simulink model "fir_multi_test"  (Simulink 7.8)
settings: Solver=ode45  StartTime=0.0  StopTime=15e-4  RelTol=1e-3
undefined symbols (not defined in the file): calc_dds_freq, Fs_adc, Fs_adc_image, xlipgetpartsetting
libraries: xbsIndex_r4 x24
settings Model: Creator=lucas.russo  LastModifiedBy=lucas.russo

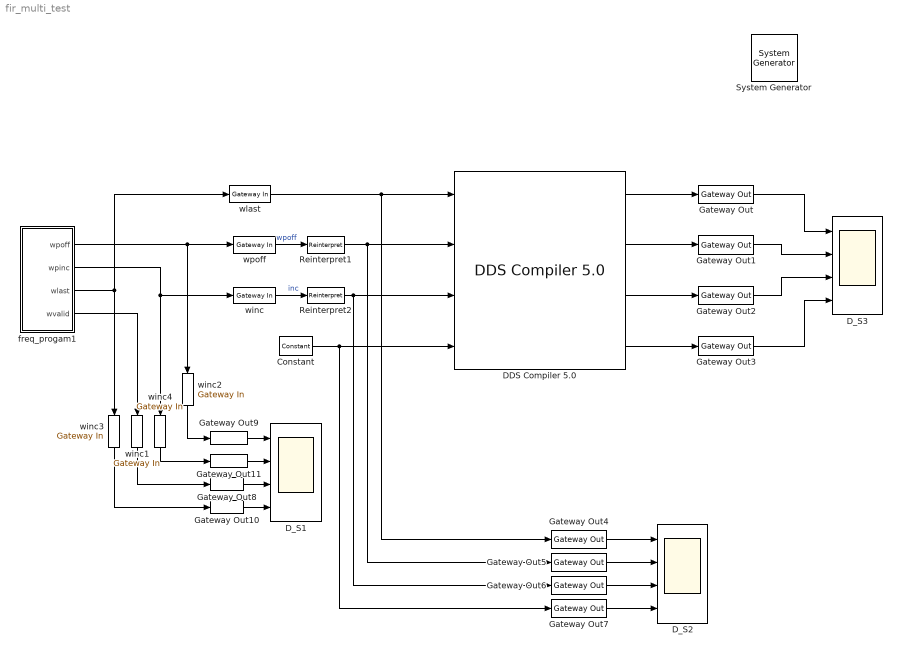
== system fir_multi_test ==
  " System Generator" : xbsIndex_r4/ System Generator  Tag=genX  xilinxfamily=virtex6  part=xc6vlx240t  speed=-1  package=ff1156  synthesis_tool=XST  clock_wrapper=Clock Enables  directory=./netlist  proj_type=Project Navigator  Synth_file=XST Defaults  Impl_file=ISE Defaults  testbench=off  simulink_period=dt_sim  sysclk_period=20  dcm_input_clock_period=10  incr_netlist=off  trim_vbits=Everywhere in SubSystem  dbl_ovrd=According to Block Masks  core_generation=According to Block Masks  run_coregen=off  deprecated_control=off  eval_field=0  block_type=sysgen
  Constant : xbsIndex_r4/Constant  const=1  gui_display_data_type=Boolean  arith_type=Boolean  n_bits=1  bin_pt=0  preci_type=Single  exp_width=8  frac_width=24  explicit_period=on  period=dt_sim  equ=P=C  opselect=C  inp2=PCIN>>17  opr=+  inp1=P  carry=CIN  dbl_ovrd=off  block_type=constant
  DDS Compiler 5.0 : xbsIndex_r4/DDS Compiler 5.0   partspresent=Phase_Generator_and_SIN_COS_LUT  dds_clock_rate=Fs_adc/1e6  channels=1  parameter_entry=Hardware_Parameters  spurious_free_dynamic_range=36  frequency_resolution=0.4  noise_shaping=Taylor_Series_Corrected  phase_width=30  output_width=24  output_selection=Sine_and_Cosine  negative_sine=on  negative_cosine=off  amplitude_mode=Unit_Circle  memory_type=Auto  optimization_goal=Auto  dsp48_use=Minimal  latency_configuration=Auto  latency=14  has_phase_out=off  has_aclken=off  has_aresetn=off  explicit_period=on  period=dt_sim  data_has_tlast=Not_Required  has_tready=on  s_phase_has_tuser=Not_Required  m_data_has_tuser=Not_Required  m_phase_has_tuser=Not_Required  s_phase_tuser_width=1  s_config_sync_mode=On_Vector  phase_increment=Programmable  output_frequency1=0  output_frequency2=0  output_frequency3=0  output_frequency4=0  output_frequency5=0  output_frequency6=0  output_frequency7=0  output_frequency8=0  output_frequency9=0  output_frequency10=0  output_frequency11=0  output_frequency12=0  output_frequency13=0  output_frequency14=0  output_frequency15=0  output_frequency16=0  pinc1='0'  pinc2='0'  pinc3='0'  pinc4='0'  pinc5='0'  pinc6='0'  pinc7='0'  pinc8='0'  pinc9='0'  pinc10='0'  pinc11='0'  pinc12='0'  pinc13='0'  pinc14='0'  pinc15='0'  pinc16='0'  phase_offset=Programmable  phase_offset_angles1=0  phase_offset_angles2=0  phase_offset_angles3=0  phase_offset_angles4=0  phase_offset_angles5=0  phase_offset_angles6=0  phase_offset_angles7=0  phase_offset_angles8=0  phase_offset_angles9=0  phase_offset_angles10=0  phase_offset_angles11=0  phase_offset_angles12=0  phase_offset_angles13=0  phase_offset_angles14=0  phase_offset_angles15=0  phase_offset_angles16=0  poff1='0'  poff2='0'  poff3='0'  poff4='0'  poff5='0'  poff6='0'  poff7='0'  poff8='0'  poff9='0'  poff10='0'  poff11='0'  poff12='0'  poff13='0'  poff14='0'  poff15='0'  poff16='0'  trim_axipin_name=on  por_mode=false  gui_behaviour=Sysgen  ip_name=DDS Compiler  ip_version=5.0  dsptool_ready=true  wrapper_available=true  port_translation_map={ 'aclken' => 'en', 'aresetn' => 'rst' }  ipcore_xco_need_fpga_part=true  ipcore_fpga_part=xlipgetpartsetting(gcb, {'virtex6', 'xc6vlx75t', '-3', 'ff784'})  ipcore_usecache=true  ipcore_useipmodelcache=true  ipcore_verbose=false  block_type=dds_compiler_v5_0
  D_S1 : Scope  NumInputPorts=4
      settings: TimeRange=0.0004  YMin=0.95~0.95~-1~0.95  YMax=1.05~1.05~1~1.05  MaxDataPoints=1000000  SampleInput=on
  D_S2 : Scope  NumInputPorts=4
      settings: TimeRange=0.0004  YMin=0.95~0.95~-1~0.95  YMax=1.05~1.05~1~1.05  SaveName=ScopeData2  MaxDataPoints=1000000  SampleInput=on
  D_S3 : Scope  NumInputPorts=4
      settings: TimeRange=0.0004  YMin=1~1~-1~1  YMax=1~1~1~1  MaxDataPoints=1000000  SampleInput=on
  Gateway Out{,1..11} (12 alike) : xbsIndex_r4/Gateway Out  inherit_from_input=on  hdl_port=on  timing_constraint=None  locs_specified=off  LOCs={}  UseAsDAC=off  DACChannel='1'  block_type=gatewayout
      settings: infoedit="Gateway out block.  Converts Xilinx fixed-point or floating-point type inputs into ouputs of type Simulink integer, single, double, or fixed point.<br><br>Hardware notes:  In hardware these blocks become top level output ports or are discarded, depending on how they are configured."
  Reinterpret1 : xbsIndex_r4/Reinterpret  force_arith_type=off  arith_type=Unsigned  force_bin_pt=on  bin_pt=30  block_type=reinterpret
  Reinterpret2 : xbsIndex_r4/Reinterpret  force_arith_type=off  arith_type=Unsigned  force_bin_pt=on  bin_pt=30  block_type=reinterpret
  freq_progam1 : Subsystem  mask(DDS Freq. Programming Stimulus){FREQ_VEC=[ Fs_adc_image ] / 1e6, Fc=Fs_adc/1e6, Pwidth=30}
      mask prompts: FREQ_VEC "Frequency Vector (MHz)"; Fc "Sample Freq (MHz)"; Pwidth "DDS Phase Width (bits)"
      mask help: This block writes the desired mixing freqencies into the programmable frequency port of the DDS.
  winc : xbsIndex_r4/Gateway In  gui_display_data_type=Fixed-point  arith_type="Signed  (2's comp)"  n_bits=30  bin_pt=0  preci_type=Single  exp_width=8  frac_width=24  quantization=Truncate  overflow=Wrap  period=dt_sim  dbl_ovrd=off  timing_constraint=None  locs_specified=off  LOCs={}  inherit_from_input=off  UseAsADC=off  ADCChannel='1'  hdl_port=on  block_type=gatewayin
      settings: infoedit="Gateway in block.  Converts inputs of type Simulink integer, single, double and fixed point to  Xilinx fixed-point or floating-point data type.<br><br>Hardware notes:  In hardware these blocks become top level input ports."
  winc1 : xbsIndex_r4/Gateway In  gui_display_data_type=Boolean  arith_type=Boolean  n_bits=30  bin_pt=0  preci_type=Single  exp_width=8  frac_width=24  quantization=Truncate  overflow=Wrap  period=dt_sim  dbl_ovrd=off  timing_constraint=None  locs_specified=off  LOCs={}  inherit_from_input=off  UseAsADC=off  ADCChannel='1'  hdl_port=on  block_type=gatewayin
      settings: infoedit="Gateway in block.  Converts inputs of type Simulink integer, single, double and fixed point to  Xilinx fixed-point or floating-point data type.<br><br>Hardware notes:  In hardware these blocks become top level input ports."
  winc2 : xbsIndex_r4/Gateway In  gui_display_data_type=Fixed-point  arith_type="Signed  (2's comp)"  n_bits=30  bin_pt=0  preci_type=Single  exp_width=8  frac_width=24  quantization=Truncate  overflow=Wrap  period=dt_sim  dbl_ovrd=off  timing_constraint=None  locs_specified=off  LOCs={}  inherit_from_input=off  UseAsADC=off  ADCChannel='1'  hdl_port=on  block_type=gatewayin
      settings: infoedit="Gateway in block.  Converts inputs of type Simulink integer, single, double and fixed point to  Xilinx fixed-point or floating-point data type.<br><br>Hardware notes:  In hardware these blocks become top level input ports."
  winc3 : xbsIndex_r4/Gateway In  gui_display_data_type=Boolean  arith_type=Boolean  n_bits=30  bin_pt=0  preci_type=Single  exp_width=8  frac_width=24  quantization=Truncate  overflow=Wrap  period=dt_sim  dbl_ovrd=off  timing_constraint=None  locs_specified=off  LOCs={}  inherit_from_input=off  UseAsADC=off  ADCChannel='1'  hdl_port=on  block_type=gatewayin
      settings: infoedit="Gateway in block.  Converts inputs of type Simulink integer, single, double and fixed point to  Xilinx fixed-point or floating-point data type.<br><br>Hardware notes:  In hardware these blocks become top level input ports."
  winc4 : xbsIndex_r4/Gateway In  gui_display_data_type=Fixed-point  arith_type="Signed  (2's comp)"  n_bits=30  bin_pt=0  preci_type=Single  exp_width=8  frac_width=24  quantization=Truncate  overflow=Wrap  period=dt_sim  dbl_ovrd=off  timing_constraint=None  locs_specified=off  LOCs={}  inherit_from_input=off  UseAsADC=off  ADCChannel='1'  hdl_port=on  block_type=gatewayin
      settings: infoedit="Gateway in block.  Converts inputs of type Simulink integer, single, double and fixed point to  Xilinx fixed-point or floating-point data type.<br><br>Hardware notes:  In hardware these blocks become top level input ports."
  wlast : xbsIndex_r4/Gateway In  gui_display_data_type=Boolean  arith_type=Boolean  n_bits=1  bin_pt=0  preci_type=Single  exp_width=8  frac_width=24  quantization=Truncate  overflow=Wrap  period=dt_sim  dbl_ovrd=off  timing_constraint=None  locs_specified=off  LOCs={}  inherit_from_input=off  UseAsADC=off  ADCChannel='1'  hdl_port=on  block_type=gatewayin
      settings: infoedit="Gateway in block.  Converts inputs of type Simulink integer, single, double and fixed point to  Xilinx fixed-point or floating-point data type.<br><br>Hardware notes:  In hardware these blocks become top level input ports."
  wpoff : xbsIndex_r4/Gateway In  gui_display_data_type=Fixed-point  arith_type="Signed  (2's comp)"  n_bits=30  bin_pt=0  preci_type=Single  exp_width=8  frac_width=24  quantization=Truncate  overflow=Wrap  period=dt_sim  dbl_ovrd=off  timing_constraint=None  locs_specified=off  LOCs={}  inherit_from_input=off  UseAsADC=off  ADCChannel='1'  hdl_port=on  block_type=gatewayin
      settings: infoedit="Gateway in block.  Converts inputs of type Simulink integer, single, double and fixed point to  Xilinx fixed-point or floating-point data type.<br><br>Hardware notes:  In hardware these blocks become top level input ports."
  wires:
  winc/1 -> Reinterpret2/1  "inc"
  Constant/1 -> Gateway Out7/1, DDS Compiler 5.0/4
  wpoff/1 -> Reinterpret1/1  "wpoff"
  DDS Compiler 5.0/4 -> Gateway Out3/1
  DDS Compiler 5.0/3 -> Gateway Out2/1
  DDS Compiler 5.0/2 -> Gateway Out1/1
  DDS Compiler 5.0/1 -> Gateway Out/1
  Gateway Out/1 -> D_S3/1
  Gateway Out1/1 -> D_S3/2
  Gateway Out2/1 -> D_S3/3
  Gateway Out3/1 -> D_S3/4
  freq_progam1/2(wpinc) -> winc/1, winc4/1
  freq_progam1/1(wpoff) -> wpoff/1, winc2/1
  freq_progam1/3(wlast) -> wlast/1, winc3/1
  wlast/1 -> DDS Compiler 5.0/1, Gateway Out4/1
  freq_progam1/4(wvalid) -> winc1/1
  Gateway Out4/1 -> D_S2/1
  Gateway Out5/1 -> D_S2/2
  Gateway Out6/1 -> D_S2/3
  Gateway Out7/1 -> D_S2/4
  Reinterpret1/1 -> DDS Compiler 5.0/2, Gateway Out5/1
  Reinterpret2/1 -> DDS Compiler 5.0/3, Gateway Out6/1
  winc1/1 -> Gateway Out8/1
  Gateway Out8/1 -> D_S1/3
  winc2/1 -> Gateway Out9/1
  Gateway Out9/1 -> D_S1/1
  winc3/1 -> Gateway Out10/1
  Gateway Out10/1 -> D_S1/4
  Gateway Out11/1 -> D_S1/2
  winc4/1 -> Gateway Out11/1

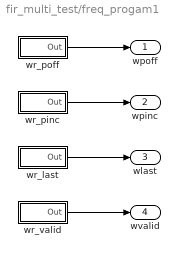
== system fir_multi_test/freq_progam1 ==
  wr_last : Subsystem
  wr_pinc : Subsystem
  wr_poff : Subsystem
  wr_valid : Subsystem
  wpoff : Outport
  wpinc : Outport  Port=2
  wlast : Outport  Port=3
  wvalid : Outport  Port=4
  wires:
  wr_last/1(Out) -> wlast/1
  wr_poff/1(Out) -> wpoff/1
  wr_pinc/1(Out) -> wpinc/1
  wr_valid/1(Out) -> wvalid/1

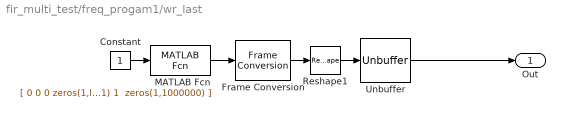
== system fir_multi_test/freq_progam1/wr_last ==
  Constant : Constant
  Frame Conversion : FrameConversion
  MATLAB Fcn : MATLABFcn  MATLABFcn="[ 0 0 0 zeros(1,length(FREQ_VEC)-1) 1  zeros(1,1000000) ]"  Output1D=off
  Reshape1 : Reshape  OutputDimensionality=Column vector (2-D)
  Unbuffer : Unbuffer
  Out : Outport
  wires:
  Constant/1 -> MATLAB Fcn/1
  MATLAB Fcn/1 -> Frame Conversion/1
  Reshape1/1 -> Unbuffer/1
  Frame Conversion/1 -> Reshape1/1
  Unbuffer/1 -> Out/1

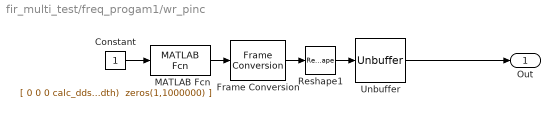
== system fir_multi_test/freq_progam1/wr_pinc ==
  Constant : Constant
  Frame Conversion : FrameConversion
  MATLAB Fcn : MATLABFcn  MATLABFcn="[ 0 0 0 calc_dds_freq(Fc, FREQ_VEC , Pwidth)  zeros(1,1000000) ]"  Output1D=off
  Reshape1 : Reshape  OutputDimensionality=Column vector (2-D)
  Unbuffer : Unbuffer
  Out : Outport
  wires:
  Unbuffer/1 -> Out/1
  Frame Conversion/1 -> Reshape1/1
  Reshape1/1 -> Unbuffer/1
  MATLAB Fcn/1 -> Frame Conversion/1
  Constant/1 -> MATLAB Fcn/1

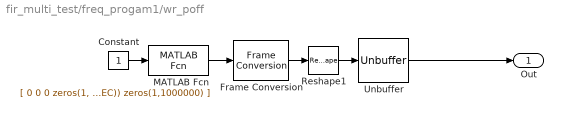
== system fir_multi_test/freq_progam1/wr_poff ==
  Constant : Constant
  Frame Conversion : FrameConversion
  MATLAB Fcn : MATLABFcn  MATLABFcn="[ 0 0 0 zeros(1,  length(FREQ_VEC)) zeros(1,1000000) ]"  Output1D=off
  Reshape1 : Reshape  OutputDimensionality=Column vector (2-D)
  Unbuffer : Unbuffer
  Out : Outport
  wires:
  Unbuffer/1 -> Out/1
  Frame Conversion/1 -> Reshape1/1
  Reshape1/1 -> Unbuffer/1
  MATLAB Fcn/1 -> Frame Conversion/1
  Constant/1 -> MATLAB Fcn/1

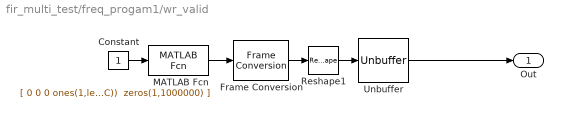
== system fir_multi_test/freq_progam1/wr_valid ==
  Constant : Constant
  Frame Conversion : FrameConversion
  MATLAB Fcn : MATLABFcn  MATLABFcn="[ 0 0 0 ones(1,length(FREQ_VEC))  zeros(1,1000000) ]"  Output1D=off
  Reshape1 : Reshape  OutputDimensionality=Column vector (2-D)
  Unbuffer : Unbuffer
  Out : Outport
  wires:
  Unbuffer/1 -> Out/1
  Frame Conversion/1 -> Reshape1/1
  Reshape1/1 -> Unbuffer/1
  MATLAB Fcn/1 -> Frame Conversion/1
  Constant/1 -> MATLAB Fcn/1
